simulink model "control"  (R2016b)
settings: Solver=FixedStepAuto  StartTime=0.0  StopTime=10.0  RelTol=1e-3  EnableMultiTasking=on
undefined symbols (not defined in the file): Rot
libraries: legoev3lib x4, simulink x1
settings Model: ExtModeTrigDuration=2  Creator=Nexel  LastModifiedBy=Nexel
settings SolverCC: PositivePriorityOrder=on
settings OptimizationCC: MaxStackSize=64
settings DebuggingCC: ParameterTunabilityLossMsg=error
settings HardwareCC: ProdBitPerPointer=32  ProdBitPerSizeT=32  ProdBitPerPtrDiffT=32  ProdLargestAtomicInteger=Long  ProdWordSize=32  ProdHWDeviceType=ARM Compatible->ARM 9
settings RTWCC: SystemTargetFile=ert.tlc  HardwareBoard=LEGO MINDSTORMS EV3  TLCOptions="-aInlineSetEventsForThisBaseRateFcn=TLC_FALSE -aSuppressMultiTaskScheduler=TLC_FALSE  -aRateBasedStepFcn=0"  TemplateMakefile=ert_default_tmf  Description=Embedded Coder  GenerateReport=on  Toolchain=Sourcery G++ Lite v2009q3  IncludeHyperlinkInReport=on  LaunchReport=on  GenerateTraceInfo=on  GenerateTraceReport=on  GenerateTraceReportSl=on  GenerateTraceReportSf=on  GenerateTraceReportEml=on
settings CodeAppCC: ForceParamTrailComments=on  IgnoreCustomStorageClasses=off  OperatorAnnotations=on  SimulinkDataObjDesc=on  SFDataObjDesc=on  MATLABFcnDesc=on  InsertBlockDesc=on  MATLABSourceComments=on
settings ERTTargetCC: SupportContinuousTime=on  SupportVariableSizeSignals=on

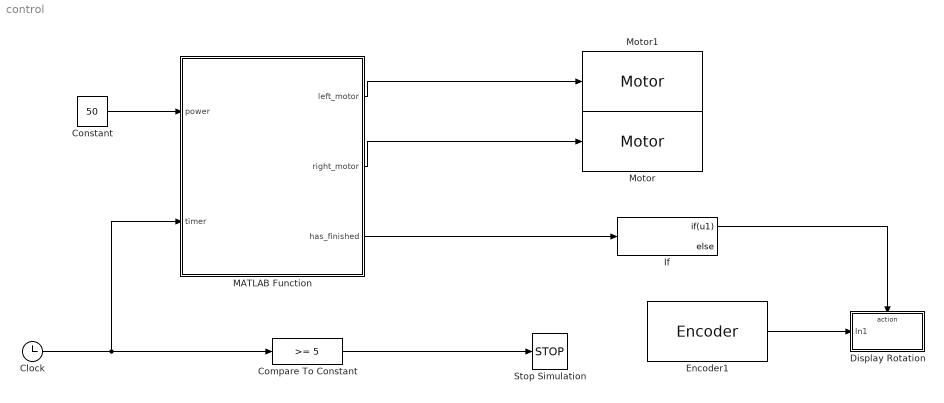
== system control ==
  Clock : Clock
      settings: Decimation=1000
  Compare To Constant : simulink/Logic and Bit Operations/Compare To Constant  relop=>=  const=5  OutDataTypeStr=boolean
  Constant : Constant  Value=50
  "Display Rotation " : Subsystem  TreatAsAtomicUnit=on
  Encoder1 : legoev3lib/Encoder  portNumber=B  opMode=No reset  sampleTime=0.1
  If : If  IfExpression=u1
  MATLAB Function : MATLAB Function  TreatAsAtomicUnit=on
  Motor : legoev3lib/Motor  sportNumber=B  sstopAction=Brake
  Motor1 : legoev3lib/Motor  sportNumber=C  sstopAction=Brake
  Stop Simulation : Stop
  wires:
  Compare To Constant/1 -> Stop Simulation/1
  Clock/1 -> MATLAB Function/2(timer), Compare To Constant/1
  Encoder1/1 -> "Display Rotation "/1(In1)
  Constant/1 -> MATLAB Function/1(power)
  MATLAB Function/2(right_motor) -> Motor/1
  MATLAB Function/1(left_motor) -> Motor1/1
  MATLAB Function/3(has_finished) -> If/1
  If/1 -> "Display Rotation "/Action

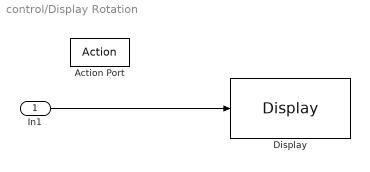
== system control/Display Rotation  ==
  In1 : Inport
  Action Port : ActionPort  ActionType=then
  Display : legoev3lib/Display  slcdStr=Rot:  slcdLine=2  slcdFormat=Decimal
  wires:
  In1/1 -> Display/1

== matlab function control/MATLAB Function ==
  data: left_motor output; power input; right_motor output; has_finished output; timer input
function [left_motor, right_motor, has_finished] = fcn(power, timer)
     %#codegen
     if(timer < 2)
         has_finished = false;
         left_motor = power;
         right_motor = power;
     else
         left_motor = 0;
         right_motor = 0;
         has_finished = true;
     end      
end
